simulink model "cascadepid"  (R2022b)
settings: Solver=VariableStepAuto  StartTime=0.0  StopTime=4.8931  FixedStep=0.048931  RelTol=1e-3
model workspace (MAT data in the model file):
  Kt = Simulink.Parameter
  Kt.DataType = 'auto'
  Kt.Complexity = 'real'
  Kt.Dimensions = [0 0]
settings Model: Creator=AD  LastModifiedBy=AD

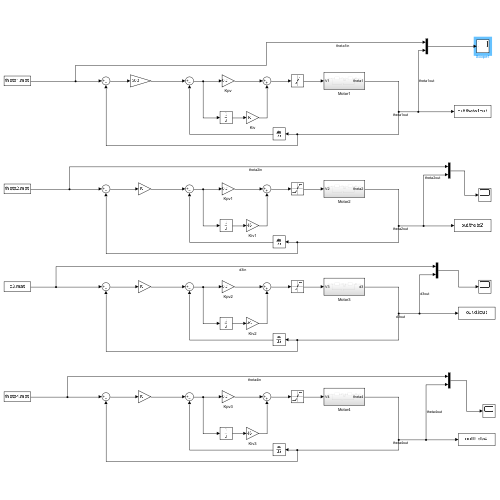
[thumbnail: Simulink's stored preview of the top-level diagram]
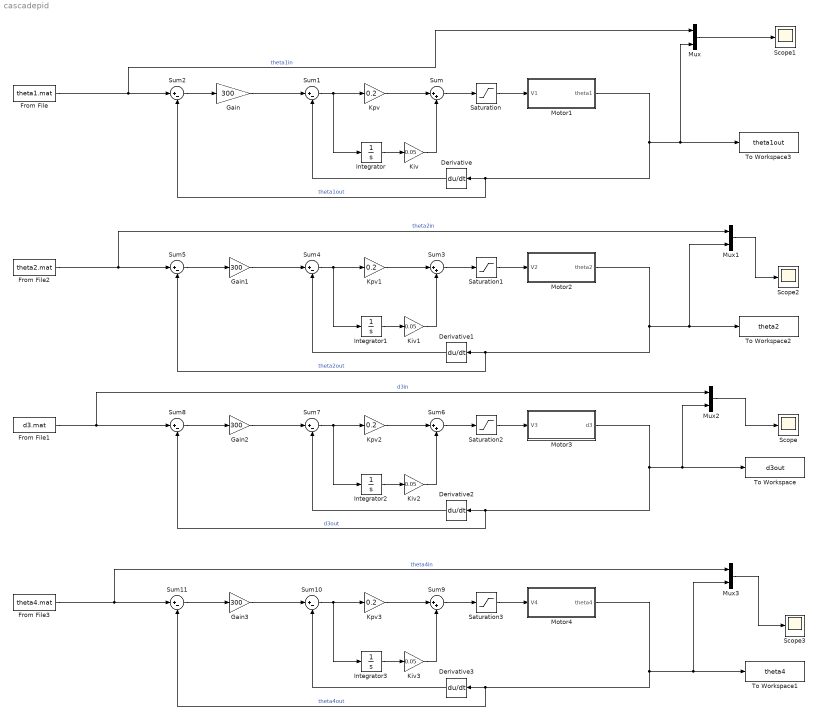
== system cascadepid ==
  Derivative{,1..3} (4 alike) : Derivative
  From File : FromFile  FileName=theta1.mat  SampleTime=0
  From File1 : FromFile  FileName=d3.mat  SampleTime=0
  From File2 : FromFile  FileName=theta2.mat  SampleTime=0
  From File3 : FromFile  FileName=theta4.mat  SampleTime=0
  Gain{,1..3} (4 alike) : Gain  Gain=300
  Integrator{,1..3} (4 alike) : Integrator
  Kiv{,1..3} (4 alike) : Gain  Gain=0.05
  Kpv{,1..3} (4 alike) : Gain  Gain=0.2
  Motor1 : Subsystem
  Motor2 : Subsystem
  Motor3 : Subsystem
  Motor4 : Subsystem
  Mux{,1..3} (4 alike) : Mux  Inputs=2
  Saturation{,1..3} (4 alike) : Saturate  UpperLimit=300  LowerLimit=-300
  Scope{,1..3} (4 alike) : Scope
  Sum{,3,6,9} (4 alike) : Sum  Inputs=|++
  Sum{1..2,4..5,7..8,10..11} (8 alike) : Sum  Inputs=|+-
  To Workspace : ToWorkspace  VariableName=d3out  SampleTime=-1
  To Workspace1 : ToWorkspace  VariableName=theta4  SampleTime=-1
  To Workspace2 : ToWorkspace  VariableName=theta2  SampleTime=-1
  To Workspace3 : ToWorkspace  VariableName=theta1out  SampleTime=-1
  wires:
  Saturation/1 -> Motor1/1(V1)
  Sum/1 -> Saturation/1
  Kpv/1 -> Sum/1
  Integrator/1 -> Kiv/1
  Kiv/1 -> Sum/2
  Sum1/1 -> Integrator/1, Kpv/1
  Derivative/1 -> Sum1/2
  Gain/1 -> Sum1/1
  Sum2/1 -> Gain/1
  Motor1/1(theta1) -> Mux/2, To Workspace3/1, Sum2/2, Derivative/1  "theta1out"
  From File/1 -> Mux/1, Sum2/1  "theta1in"
  Sum5/1 -> Gain1/1
  Motor2/1(theta2) -> Mux1/2, To Workspace2/1, Sum5/2, Derivative1/1  "theta2out"
  Gain1/1 -> Sum4/1
  Kpv1/1 -> Sum3/1
  Saturation1/1 -> Motor2/1(V2)
  Kiv1/1 -> Sum3/2
  Sum3/1 -> Saturation1/1
  Derivative1/1 -> Sum4/2
  Integrator1/1 -> Kiv1/1
  Sum4/1 -> Integrator1/1, Kpv1/1
  Sum8/1 -> Gain2/1
  Motor3/1(d3) -> Mux2/2, To Workspace/1, Sum8/2, Derivative2/1  "d3out"
  Gain2/1 -> Sum7/1
  Kpv2/1 -> Sum6/1
  Saturation2/1 -> Motor3/1(V3)
  Kiv2/1 -> Sum6/2
  Sum6/1 -> Saturation2/1
  Derivative2/1 -> Sum7/2
  Integrator2/1 -> Kiv2/1
  Sum7/1 -> Integrator2/1, Kpv2/1
  Sum11/1 -> Gain3/1
  Motor4/1(theta4) -> Mux3/2, To Workspace1/1, Sum11/2, Derivative3/1  "theta4out"
  Gain3/1 -> Sum10/1
  Kpv3/1 -> Sum9/1
  Saturation3/1 -> Motor4/1(V4)
  Kiv3/1 -> Sum9/2
  Sum9/1 -> Saturation3/1
  Derivative3/1 -> Sum10/2
  Integrator3/1 -> Kiv3/1
  Sum10/1 -> Integrator3/1, Kpv3/1
  From File1/1 -> Mux2/1, Sum8/1  "d3in"
  From File3/1 -> Mux3/1, Sum11/1  "theta4in"
  From File2/1 -> Mux1/1, Sum5/1  "theta2in"
  Mux/1 -> Scope1/1
  Mux1/1 -> Scope2/1
  Mux2/1 -> Scope/1
  Mux3/1 -> Scope3/1

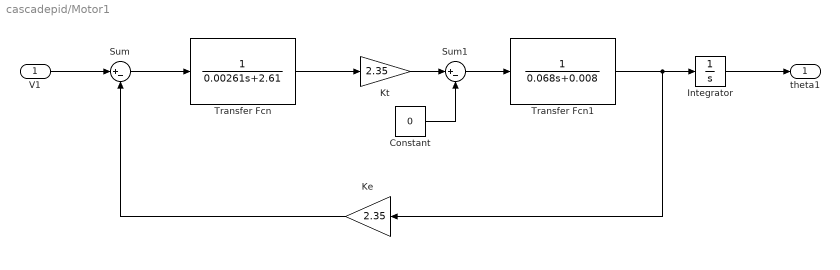
== system cascadepid/Motor1 ==
  V1 : Inport
  Constant : Constant  Value=0
  Integrator : Integrator
  Ke : Gain  Gain=2.35
  Kt : Gain  Gain=2.35
  Sum : Sum  Inputs=|+-
  Sum1 : Sum  Inputs=|+-
  Transfer Fcn : TransferFcn  Numerator=[0 1]  Denominator=[0.00261 2.61]
  Transfer Fcn1 : TransferFcn  Numerator=[0 1]  Denominator=[0.068 0.008]
  theta1 : Outport
  wires:
  Sum/1 -> Transfer Fcn/1
  Transfer Fcn/1 -> Kt/1
  Kt/1 -> Sum1/1
  Sum1/1 -> Transfer Fcn1/1
  Integrator/1 -> theta1/1
  Transfer Fcn1/1 -> Ke/1, Integrator/1
  Ke/1 -> Sum/2
  Constant/1 -> Sum1/2
  V1/1 -> Sum/1

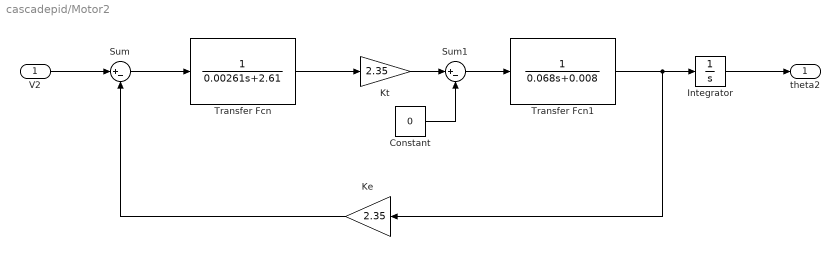
== system cascadepid/Motor2 ==
  V2 : Inport
  Constant : Constant  Value=0
  Integrator : Integrator
  Ke : Gain  Gain=2.35
  Kt : Gain  Gain=2.35
  Sum : Sum  Inputs=|+-
  Sum1 : Sum  Inputs=|+-
  Transfer Fcn : TransferFcn  Numerator=[0 1]  Denominator=[0.00261 2.61]
  Transfer Fcn1 : TransferFcn  Numerator=[0 1]  Denominator=[0.068 0.008]
  theta2 : Outport
  wires:
  Sum/1 -> Transfer Fcn/1
  Transfer Fcn/1 -> Kt/1
  Kt/1 -> Sum1/1
  Sum1/1 -> Transfer Fcn1/1
  Integrator/1 -> theta2/1
  Transfer Fcn1/1 -> Ke/1, Integrator/1
  Ke/1 -> Sum/2
  Constant/1 -> Sum1/2
  V2/1 -> Sum/1

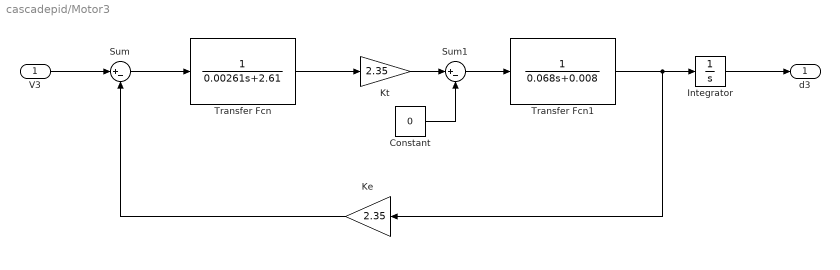
== system cascadepid/Motor3 ==
  V3 : Inport
  Constant : Constant  Value=0
  Integrator : Integrator
  Ke : Gain  Gain=2.35
  Kt : Gain  Gain=2.35
  Sum : Sum  Inputs=|+-
  Sum1 : Sum  Inputs=|+-
  Transfer Fcn : TransferFcn  Numerator=[0 1]  Denominator=[0.00261 2.61]
  Transfer Fcn1 : TransferFcn  Numerator=[0 1]  Denominator=[0.068 0.008]
  d3 : Outport
  wires:
  Sum/1 -> Transfer Fcn/1
  Transfer Fcn/1 -> Kt/1
  Kt/1 -> Sum1/1
  Sum1/1 -> Transfer Fcn1/1
  Integrator/1 -> d3/1
  Transfer Fcn1/1 -> Ke/1, Integrator/1
  Ke/1 -> Sum/2
  Constant/1 -> Sum1/2
  V3/1 -> Sum/1

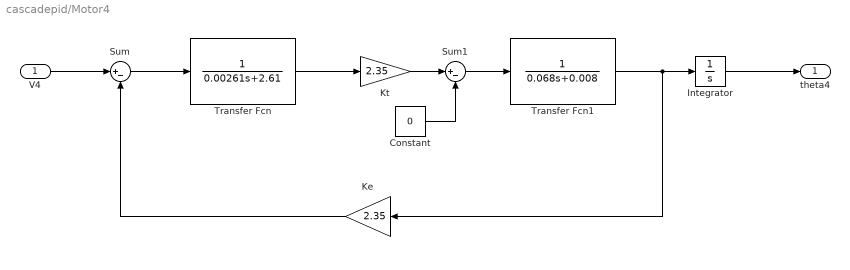
== system cascadepid/Motor4 ==
  V4 : Inport
  Constant : Constant  Value=0
  Integrator : Integrator
  Ke : Gain  Gain=2.35
  Kt : Gain  Gain=2.35
  Sum : Sum  Inputs=|+-
  Sum1 : Sum  Inputs=|+-
  Transfer Fcn : TransferFcn  Numerator=[0 1]  Denominator=[0.00261 2.61]
  Transfer Fcn1 : TransferFcn  Numerator=[0 1]  Denominator=[0.068 0.008]
  theta4 : Outport
  wires:
  Sum/1 -> Transfer Fcn/1
  Transfer Fcn/1 -> Kt/1
  Kt/1 -> Sum1/1
  Sum1/1 -> Transfer Fcn1/1
  Integrator/1 -> theta4/1
  Transfer Fcn1/1 -> Ke/1, Integrator/1
  Ke/1 -> Sum/2
  Constant/1 -> Sum1/2
  V4/1 -> Sum/1
